simulink model "master"  (R2020b)
settings: Solver=VariableStepAuto  StartTime=0.0  StopTime=752  RelTol=1e-3
values from neighbouring files (symbols this model uses):
  a = [a;0]    [init.m]
  h = load('Hoehe.txt')    [Projektskript.m]    (also in init.m)
  rrad = 0.3    [Projektskript.m]    (also in init.m)
  s = cumtrapz(v)    [init.m]
  s_real_cum = cumsum(s_real)    [init.m]
  v = load('Geschwindigkeit.txt')    [Projektskript.m]    (also in init.m)
  v_real = gradient(s_real_cum)    [init.m]
libraries: simulink x1, Motor_Power_v2 x1, air_resistance x1, Gradiantel_Force x1, friction_resistance x1, rotation_resistance x1, trans_resistance x1, gear x1
Description:
  | ----------------Fahrsimulation  eines Elektroautos-----------
  | 
  | Das Modell simuliert auf Grundlage der Daten aus dem Matlab Skript die Fahrt über einem vorgegebenem Höhen- und Streckenverlauf.
  | Durch eine Simulationszeit getriggert- wird zu jedem Simulationsschritt die effektive Leistung berechnet. Als Zwischenschritte muss dafür über die wirkende Kräfte zunächst Drehmoment und Winkelgeschwindigkeiten am Rad bestimmt werden. Anschließend wird über die entsprechende Getriebeübersetzung Winkelgeschwindigkeit und Drehmoment am Motor berechnet. Letzlich kann wird unter Berücksi chtigung der Kenngrößen des Motors sowie unter Berücksichtigung weiterer Verbraucher die Effektivleistung berechnet.
settings Model: PacingRate=18  Creator=Vanessa Weiß, Jonas Eckert, Jan Bantle  LastModifiedBy=Johnathy

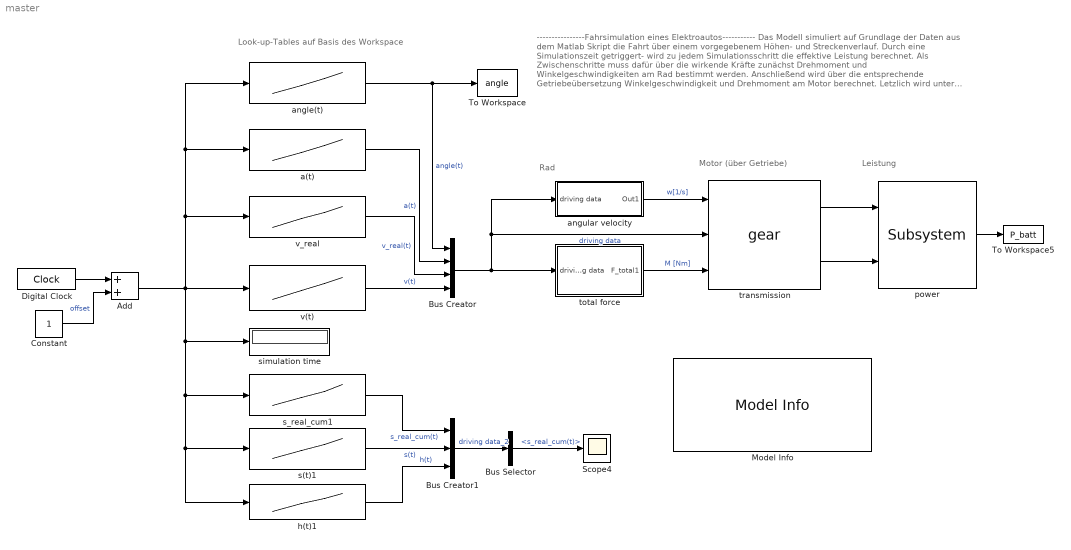
== system master ==
  note: Leistung
  note: Motor (über Getriebe)
  note: Rad
  note: Look-up-Tables auf Basis des Workspace
  note: ----------------Fahrsimulation eines Elektroautos-----------
      |
      | Das Modell simuliert auf Grundlage der Daten aus dem Matlab Skript die Fahrt über einem vorgegebenem Höhen- und Streckenverlauf.
      | Durch eine Simulationszeit getriggert- wird zu jedem Simulationsschritt die effektive Leistung berechnet. Als Zwischenschritte muss dafür über die wirkende Kräfte zunächst Drehmoment und Winkelgeschwindigkeiten am Rad bestimmt werden. Anschließend wird über die entsprechende Getriebeübersetzung Winkelgeschwindigkeit und Drehmoment am Motor berechnet. Letzlich wird unter Berücksichtigung der Kenngrößen des Motors sowie weiterer Verbraucher die Effektivleistung berechnet.
      | Sämtliche Ergebnisse werden in den Matlab Workspace geladen und dort weiter ausgewertet.
  Add : Sum
  Bus Creator : BusCreator  Inputs=4
  Bus Creator1 : BusCreator  Inputs=3
  Bus Selector : BusSelector  OutputSignals=s_real_cum(t)
  Constant : Constant
  Digital Clock : DigitalClock
  Model Info : simulink/Model-Wide Utilities/Model Info  Frame=off  DisplayStringWithTags=|  HorizontalTextAlignment=Left  LeftAlignmentValue=0.02
      | Model Info
      | Creator: 
      | %<Creator>
      | Model Verison: 
      | %<ModelVersion>
      | Last modified: 
      | %<LastModificationDate>
      | Last Modification:
      | %<LastModifiedBy>
  Scope4 : Scope
  To Workspace : ToWorkspace  VariableName=angle  SampleTime=-1
  To Workspace5 : ToWorkspace  VariableName=P_batt  SampleTime=-1
  a(t) : Lookup_n-D  NumberOfTableDimensions=1  BreakpointsForDimension1=t  BreakpointsForDimension3=[5, 7]  Table=a  InternalRulePriority=Speed  RndMeth=Simplest  InputSameDT=on
  "angle(t) " : Lookup_n-D  NumberOfTableDimensions=1  BreakpointsForDimension1=t  BreakpointsForDimension3=[5, 7]  Table=angle  InternalRulePriority=Speed  RndMeth=Simplest  InputSameDT=on
  angular velocity : Subsystem
  h(t)1 : Lookup_n-D  NumberOfTableDimensions=1  BreakpointsForDimension1=t  BreakpointsForDimension3=[5, 7]  Table=h  InternalRulePriority=Speed  RndMeth=Simplest  InputSameDT=on
  power : Motor_Power_v2/Subsystem  SystemSampleTime=-1  VariantActivationTime=update diagram  Latency=0  AutoFrameSizeCalculation=off
  s(t)1 : Lookup_n-D  NumberOfTableDimensions=1  BreakpointsForDimension1=t  BreakpointsForDimension3=[5, 7]  Table=s  InternalRulePriority=Speed  RndMeth=Simplest  InputSameDT=on
  s_real_cum1 : Lookup_n-D  NumberOfTableDimensions=1  BreakpointsForDimension1=t  BreakpointsForDimension3=[5, 7]  Table=s_real_cum  InternalRulePriority=Speed  RndMeth=Simplest  InputSameDT=on
  simulation time : Display
  total force : Subsystem
  "transmission " : gear/gear  small_gear=12.5  big_gear=5
  v(t) : Lookup_n-D  NumberOfTableDimensions=1  BreakpointsForDimension1=t  BreakpointsForDimension3=[5, 7]  Table=v  InternalRulePriority=Speed  RndMeth=Simplest  InputSameDT=on
  v_real : Lookup_n-D  NumberOfTableDimensions=1  BreakpointsForDimension1=t  BreakpointsForDimension3=[5, 7]  Table=v_real  InternalRulePriority=Speed  RndMeth=Simplest  InputSameDT=on
  wires:
  Bus Creator/1 -> angular velocity/1(driving data), "transmission "/2, total force/1(driving data)  "driving data"
  v(t)/1 -> Bus Creator/4  "v(t)"
  v_real/1 -> Bus Creator/3  "v_real(t)"
  "angle(t) "/1 -> Bus Creator/1, To Workspace/1  "angle(t)"
  angular velocity/1(Out1) -> "transmission "/1  "w[1/s]"
  "transmission "/1 -> power/1
  "transmission "/2 -> power/2
  Constant/1 -> Add/2  "offset"
  Digital Clock/1 -> Add/1
  Add/1 -> "angle(t) "/1, a(t)/1, v_real/1, v(t)/1, simulation time/1, s_real_cum1/1, s(t)1/1, h(t)1/1
  total force/1(F_total1) -> "transmission "/3  "M [Nm]"
  h(t)1/1 -> Bus Creator1/3  "h(t)"
  s_real_cum1/1 -> Bus Creator1/1  "s_real_cum(t)"
  s(t)1/1 -> Bus Creator1/2  "s(t)"
  Bus Creator1/1 -> Bus Selector/1  "driving data_2"
  Bus Selector/1 -> Scope4/1  "<s_real_cum(t)>"
  a(t)/1 -> Bus Creator/2  "a(t)"
  power/1 -> To Workspace5/1

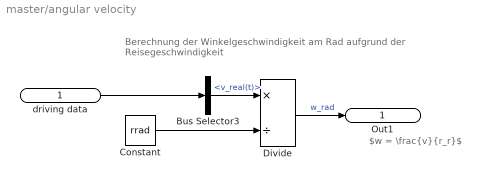
== system master/angular velocity ==
  note: $w = \frac{v}{r_r}$
  note: Berechnung der Winkelgeschwindigkeit am Rad aufgrund der
      | Reisegeschwindigkeit
  driving data : Inport
  Bus Selector3 : BusSelector  OutputSignals=v_real(t)
  Constant : Constant  Value=rrad
  Divide : Product  Inputs=*/
  Out1 : Outport
  wires:
  Bus Selector3/1 -> Divide/1  "<v_real(t)>"
  Divide/1 -> Out1/1  "w_rad"
  Constant/1 -> Divide/2
  driving data/1 -> Bus Selector3/1

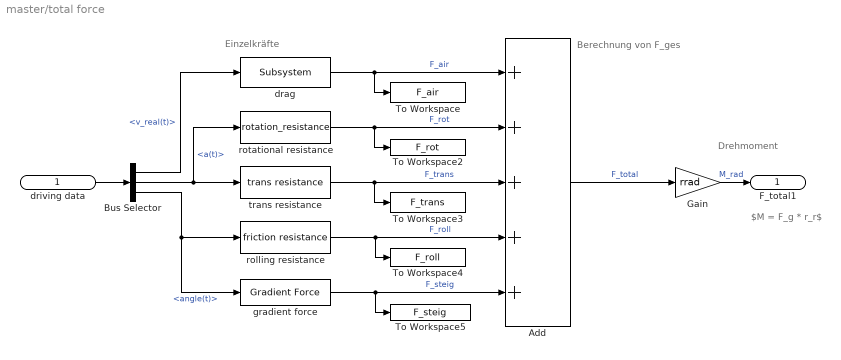
== system master/total force ==
  note: Drehmoment
  note: $M = F_g * r_r$
  note: Berechnung
      | von F_ges
  note: Einzelkräfte
  driving data : Inport
  Add : Sum  Inputs=+++++
  Bus Selector : BusSelector  OutputSignals=v_real(t),a(t),angle(t)
  Gain : Gain  Gain=rrad
  To Workspace : ToWorkspace  VariableName=F_air  SampleTime=-1
  To Workspace2 : ToWorkspace  VariableName=F_rot  SampleTime=-1
  To Workspace3 : ToWorkspace  VariableName=F_trans  SampleTime=-1
  To Workspace4 : ToWorkspace  VariableName=F_roll  SampleTime=-1
  To Workspace5 : ToWorkspace  VariableName=F_steig  SampleTime=-1
  drag : air_resistance/Subsystem  SystemSampleTime=-1  VariantActivationTime=update diagram  Latency=0  AutoFrameSizeCalculation=off
  gradient force : Gradiantel_Force/Gradient Force  SystemSampleTime=-1  VariantActivationTime=update diagram  Latency=0  AutoFrameSizeCalculation=off
  "rolling resistance " : friction_resistance/friction resistance   SystemSampleTime=-1  VariantActivationTime=update diagram  Latency=0  AutoFrameSizeCalculation=off
  rotational resistance : rotation_resistance/rotation_resistance  SystemSampleTime=-1  VariantActivationTime=update diagram  Latency=0  AutoFrameSizeCalculation=off
  trans resistance : trans_resistance/trans resistance  SystemSampleTime=-1  VariantActivationTime=update diagram  Latency=0  AutoFrameSizeCalculation=off
  F_total1 : Outport
  wires:
  drag/1 -> To Workspace/1, Add/1  "F_air"
  Bus Selector/1 -> drag/1  "<v_real(t)>"
  Bus Selector/2 -> rotational resistance/1, trans resistance/1  "<a(t)>"
  rotational resistance/1 -> To Workspace2/1, Add/2  "F_rot"
  trans resistance/1 -> To Workspace3/1, Add/3  "F_trans"
  "rolling resistance "/1 -> Add/4, To Workspace4/1  "F_roll"
  gradient force/1 -> To Workspace5/1, Add/5  "F_steig"
  Add/1 -> Gain/1  "F_total"
  Gain/1 -> F_total1/1  "M_rad"
  Bus Selector/3 -> gradient force/1, "rolling resistance "/1  "<angle(t)>"
  driving data/1 -> Bus Selector/1
